simulink model "cauchyFuncs"  (R2021a)
settings: Solver=VariableStepAuto  StartTime=0.0  StopTime=10  RelTol=1e-3
libraries: mcbcontrolslib x1, simulink x1
settings Model: Creator=z_zha  LastModifiedBy=z_zha

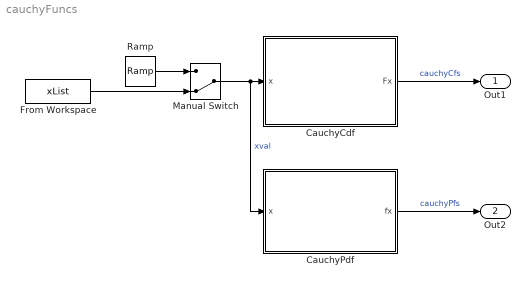
== system cauchyFuncs ==
  CauchyCdf : Subsystem  mask{ga=1, a=700, b=100}
      mask prompts: ga "Cauchy gamma value"; a "Gain factor(Range)"; b "Bias factor(Initial value)"
  CauchyPdf : Subsystem  mask{g=0.2}
      mask prompts: g "Cauchy gamma value"
      mask init:
      | ga=1;
  From Workspace : FromWorkspace  VariableName=xList
  Manual Switch : ManualSwitch  CurrentSetting=0
  Ramp : simulink/Sources/Ramp  slope=2  start=-5  InitialOutput=0
  Out1 : Outport
  Out2 : Outport  Port=2
  wires:
  Ramp/1 -> Manual Switch/1
  From Workspace/1 -> Manual Switch/2
  Manual Switch/1 -> CauchyPdf/1(x), CauchyCdf/1(x)  "xval"
  CauchyCdf/1(Fx) -> Out1/1  "cauchyCfs"
  CauchyPdf/1(fx) -> Out2/1  "cauchyPfs"

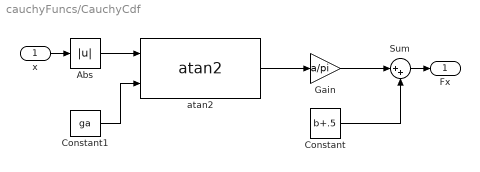
== system cauchyFuncs/CauchyCdf ==
  x : Inport
  Abs : Abs
  Constant : Constant  Value=b+.5
  Constant1 : Constant  Value=ga
  Gain : Gain  Gain=a/pi
  Sum : Sum  Inputs=|++
  atan2 : mcbcontrolslib/atan2  outputUnit=Radians
      settings: SourceProductBaseCode=MT
  Fx : Outport
  wires:
  atan2/1 -> Gain/1
  Constant1/1 -> atan2/2
  x/1 -> Abs/1
  Constant/1 -> Sum/2
  Sum/1 -> Fx/1
  Abs/1 -> atan2/1
  Gain/1 -> Sum/1

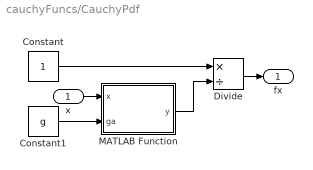
== system cauchyFuncs/CauchyPdf ==
  x : Inport
  Constant : Constant
  Constant1 : Constant  Value=g
  Divide : Product  Inputs=*/
  MATLAB Function : MATLAB Function  TreatAsAtomicUnit=on
  fx : Outport
  wires:
  Divide/1 -> fx/1
  MATLAB Function/1(y) -> Divide/2
  Constant1/1 -> MATLAB Function/2(ga)
  x/1 -> MATLAB Function/1(x)
  Constant/1 -> Divide/1

== matlab function cauchyFuncs/CauchyPdf/MATLAB Function ==
  data: x input; y output; ga input
function y = fcn(x, ga)
y = pi*(ga+x^2);
